simulink model "PWC_full"  (R2014b)
settings: Solver=ode23  StartTime=0.0  StopTime=10.0  RelTol=1e-3
libraries: commutil2 x1
settings Model: Creator=z2akhtar  LastModifiedBy=z2akhtar
settings OptimizationCC: ExpressionDepthLimit=2147483647
settings DebuggingCC: UnderspecifiedInitializationDetection=Classic  MergeDetectMultiDrivingBlocksExec=none  StateNameClashWarn=warning
settings ConfigComp: Description=Design Verifier Custom Configuration Component  DVModelCoverageObjectives=Decision  DVMaxTestCaseSteps=500  DVTestSuiteOptimization=IndividualObjectives  DVDetectActiveLogic=on

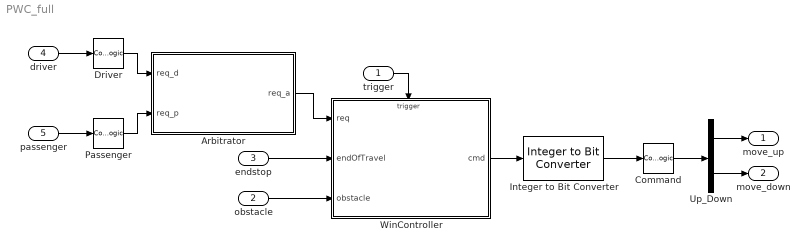
== system PWC_full ==
  trigger : Inport  OutDataTypeStr=double
  obstacle : Inport  Port=2  OutDataTypeStr=boolean
  endstop : Inport  Port=3  OutDataTypeStr=boolean
  driver : Inport  Port=4  OutDataTypeStr=boolean
  passenger : Inport  Port=5  OutDataTypeStr=boolean
  Arbitrator : MATLAB Function  TreatAsAtomicUnit=on
  Command : CombinatorialLogic  TruthTable=[0 0;0 1;1 0;0 0]
  Driver : CombinatorialLogic  TruthTable=[0;1;2;0;0;0;0;0]
  Integer to Bit Converter : commutil2/Integer to Bit Converter  nbits=2  signedInputValues=Unsigned  bitOrder=MSB first  outDtype=Inherit via internal rule
  Passenger : CombinatorialLogic  TruthTable=[0;2;1;0;0;0;0;0]
  Up_Down : Demux  Outputs=2
  WinController : Stateflow chart
  move_up : Outport  OutDataTypeStr=boolean
  move_down : Outport  Port=2  OutDataTypeStr=boolean
  wires:
  Arbitrator/1(req_a) -> WinController/1(req)
  endstop/1 -> WinController/2(endOfTravel)
  driver/1 -> Driver/1
  passenger/1 -> Passenger/1
  Passenger/1 -> Arbitrator/2(req_p)
  Command/1 -> Up_Down/1
  WinController/1(cmd) -> Integer to Bit Converter/1
  Integer to Bit Converter/1 -> Command/1
  Driver/1 -> Arbitrator/1(req_d)
  Up_Down/2 -> move_down/1
  Up_Down/1 -> move_up/1
  trigger/1 -> WinController/Trigger
  obstacle/1 -> WinController/3(obstacle)

== matlab function PWC_full/Arbitrator ==
  data: req_d input; req_a output; req_p input
function req_a = WinRqArbitrator(req_d, req_p)
%#codegen

req_a = 0;

if req_p == 0 && req_d == 0
    req_a = 0;
elseif req_p  ~= 0 && req_d == 0
    req_a = req_p;
elseif req_p == 0 && req_d ~= 0 
    req_a = req_d;
elseif req_p ~= 0 && req_d ~= 0
    req_a = 0;
end
% What if both are != stop
end

== stateflow chart PWC_full/WinController ==
  state winStates
    state Stopped
      en: cmd = 0;
      state unknownPos
      state fullyClosed
      state fullyOpen
      state partiallyOpen
      (default) -> unknownPos
      unknownPos -> partiallyOpen
      partiallyOpen -> (junction 104)
    state movingUp
      en: cmd = 2;
      state movingUpBsc
      state movingUpX
        state mux_pp
        state mux_ppo
        (default) -> mux_ppo
        mux_ppo -> mux_pp : [req ~= 4]
      (default) -> movingUpBsc
      movingUpBsc -> movingUpX [order 1] : [req == 4]
    state movingDown
      en: cmd = 1;
      state movingDownBsc
      state movingDownX
      (default) -> movingDownBsc
      movingDownBsc -> movingDownX [order 1] : [req == 3]
    state retracting
      en: cmd = 1;
    state coolDown
      en: cmd = 0;
    coolDown -> Stopped : [req == 0]
    movingUp -> fullyClosed [order 1] : [endOfTravel  == 1]
    fullyClosed -> (junction 123) [order 1] : [req == 1]
    fullyClosed -> (junction 72) [order 2] : [req==3]
    fullyOpen -> (junction 128) [order 2] : [req == 2]
    (junction 117) -> fullyOpen
    fullyOpen -> (junction 46) [order 1] : [req == 4]
    movingUpBsc -> partiallyOpen [order 2] : [(req == 0)]
    movingDownBsc -> partiallyOpen [order 2] : [req == 0]
    (junction 104) -> (junction 123) [order 2] : [req == 1]
    (junction 104) -> (junction 128) [order 1] : [req == 2]
    (junction 104) -> (junction 46) [order 4] : [req == 4]
    (junction 104) -> (junction 72) [order 3] : [req == 3]
    (junction 123) -> movingDown
    (junction 128) -> movingUp
    movingDown -> (junction 117) [order 1] : [endOfTravel]
    retracting -> (junction 117) : [endOfTravel]
    (junction 71) -> movingDownBsc
    movingUp -> (junction 71) [order 3] : [req == 1]
    movingDown -> (junction 73) [order 4] : [req == 2]
    (junction 73) -> movingUpBsc
    (junction 72) -> movingDownX
    movingUp -> (junction 72) [order 4] : [req == 3]
    movingDown -> (junction 46) [order 2] : [req == 4]
    (junction 46) -> movingUpX
    mux_pp -> (junction 39) : [obstacle == 1]
    movingDown -> coolDown [order 3] : [after(10, sec)]
    movingUp -> coolDown [order 2] : [after(10, sec)]
    (junction 39) -> retracting
  data: req input; endOfTravel input boolean; obstacle input boolean; cmd output
  events: ticks input EITHER_EDGE_EVENT
